simulink model "G_Export_V3"  (R2024b)
settings: Solver=FixedStepDiscrete  StartTime=0  StopTime=1  RelTol=1e-3
libraries: dspxfrm3 x1, dspmlti4 x1, dspsigops x1
settings Model: Creator=Lenovo  LastModifiedBy=Lenovo
settings OptimizationCC: DefaultParameterBehavior=Inlined  EnhancedBackFolding=on  PassReuseOutputArgsAs=Individual arguments  ZeroExternalMemoryAtStartup=off  ZeroInternalMemoryAtStartup=off  OptimizeBlockOrder=speed  DifferentSizesBufferReuse=on  OptimizationCustomize=off  EfficientTunableParamExpr=on
settings DebuggingCC: ParameterTunabilityLossMsg=error
settings HardwareCC: ProdBitPerPointer=32  ProdBitPerSizeT=32  ProdBitPerPtrDiffT=32  ProdLargestAtomicInteger=Long  ProdLargestAtomicFloat=Double  ProdWordSize=32  ProdHWDeviceType=ARM Compatible->ARM Cortex-M
settings SFSimCC: MATLABDynamicMemAlloc=off
settings RTWCC: Description=Embedded Coder  SystemTargetFile=ert.tlc  GenCodeOnly=on  TemplateMakefile=ert_default_tmf
settings CodeAppCC: ForceParamTrailComments=on  GenerateComments=off  IgnoreCustomStorageClasses=off  OperatorAnnotations=on  SimulinkDataObjDesc=on  SFDataObjDesc=on  InsertBlockDesc=on
settings ERTTargetCC: TargetLangStandard=C99 (ISO)  GenerateSampleERTMain=on  SupportNonFinite=off  ERTCustomFileTemplate=example_file_process.tlc

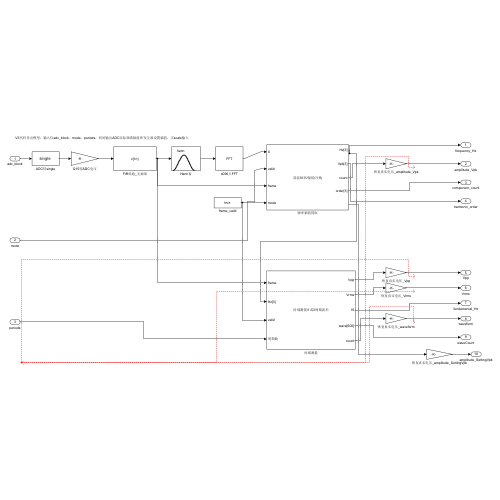
[thumbnail: Simulink's stored preview of the top-level diagram]
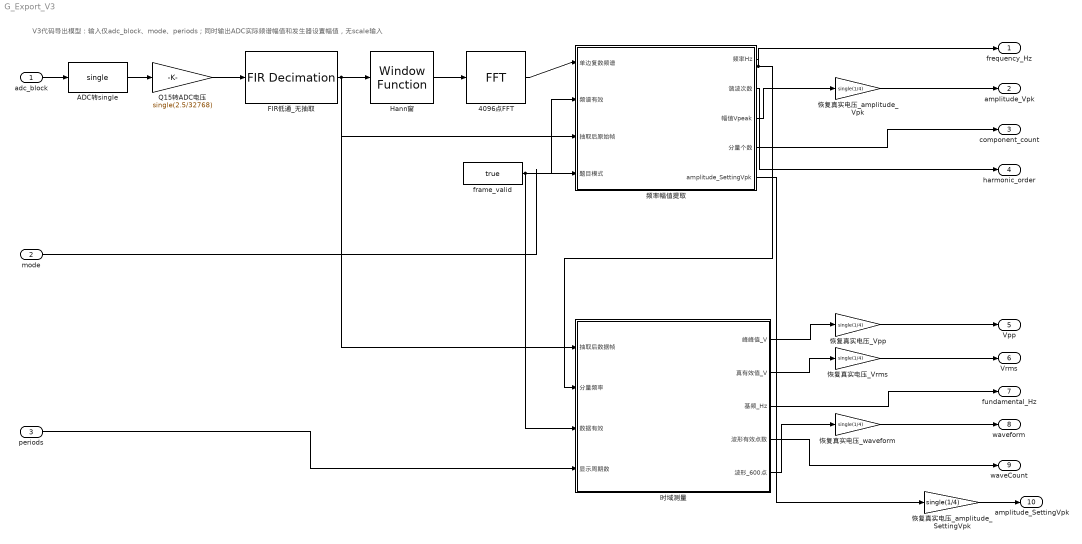
== system G_Export_V3 ==
  note: V3代码导出模型：输入仅adc_block、mode、periods；同时输出ADC实际频谱幅值和发生器设置幅值，无scale输入
  adc_block : Inport  OutDataTypeStr=int16  PortDimensions=16384
  mode : Inport  Port=2  OutDataTypeStr=uint8  PortDimensions=1
  periods : Inport  Port=3  OutDataTypeStr=uint8  PortDimensions=1
  4096点FFT : dspxfrm3/FFT  FFTImplementation=Auto  CompMethod=Table lookup  TableOpt=NEW  TableOptActive=Speed  BitRevOrder=off  Normalize=off  InheritFFTLength=on  FFTLength=64  WrapInput=on  roundingMode=Ceiling  overflowMode=off  firstCoeffDataTypeStr=Inherit: Same word length as input  firstCoeffLastDataTypeStr=Inherit: Same word length as input  outputMin=[]  outputMax=[]
  ADC转single : DataTypeConversion  OutDataTypeStr=single  SaturateOnIntegerOverflow=off  RndMeth=Floor
  FIR低通_无抽取 : dspmlti4/FIR Decimation  FilterSource=Dialog parameters  h=[-1.093832325746845e-05 -6.292254736687438e-05 -0.0001456190566409851 -0.000210121213955772 -0.0001715204318703031 5.201786070564381e-05 0.0004740892277420891 0.0009791364033496543 0.001309961916795507 0.001139443592884425 0.0002271750021134837 -0.001389645221210771 -0.00326542298539904 -0.004577381356277919 -0.004374292500219585 -0.00200400120335077 0.00242713788631572 0.00778010462815952 0.01199664830895183 0.01268492551912718 0.00806980856872996 -0.001995124150862495 -0.01536663043623436 -0.02767001830927002 -0.03323335274731441 -0.02673559895993285 -0.005096036961720372 0.03104031203495614 0.07681183656132551 0.1239468431957101 0.1627378137916923 0.184631371906325 0.184631371906325 0.1627378137916923 0.1239468431957101 0.07681183656132551 0.03104031203495614 -0.005096036961720372 -0.02673559895993285 -0.03323335274731441 -0.02767001830927002 -0.01536663043623436 -0.001995124150862495 0.00806980856872996 0.01268492551912718 0.01199664830895183 0.00778010462815952 0.00242713788631572 -0.00200400120335077 -0.004374292500219585 -0.004577381356277919 -0.00326542298539904 -0.001389645221210771 0.0002271750021134837 0.001139443592884425 0.001309961916795507 0.0009791364033496543 0.0004740892277420891 5.201786070564381e-05 -0.0001715204318703031 -0.000210121213955772 -0.0001456190566409851 -6.292254736687438e-05 -1.093832325746845e-05]  D=1  filtStruct=Direct form transposed  FilterObject=FDECIM  InputProcessing=Columns as channels (frame based)  framing=Enforce single-rate processing  AllowArbitraryInputLength=off  inputOffset=0  outputBufInitCond=0  roundingMode=Floor  overflowMode=off  firstCoeffDataTypeStr=Inherit: Same word length as input  firstCoeffMin=[]  firstCoeffMax=[]  firstCoeffLastDataTypeStr=Inherit: Same word length as input  outputDataTypeStr=Inherit: Same as accumulator  outputMin=[]  outputMax=[]  outputLastDataTypeStr=Inherit: Same as accumulator
  Hann窗 : dspsigops/Window Function  winmode=Apply window to input  wintype=Hann  sampmode=Discrete  samptime=1  N=64  Rs=50  beta=10  winsamp=Symmetric  UserWindow=hamming  OptParams=off  UserParams={'symmetric'}  dataType=double  isSigned=on  wordLen=16  udDataType=sfix(16)  fracBitsMode=Best precision  numFracBits=15  roundingMode=Floor  overflowMode=off  numSidelobes=4  sidelobeLevel=-30
  Q15转ADC电压 : Gain  Gain=single(2.5/32768)
  frame_valid : Constant  Value=true  OutDataTypeStr=boolean
  恢复真实电压_Vpp : Gain  Gain=single(1/4)
  恢复真实电压_Vrms : Gain  Gain=single(1/4)
  恢复真实电压_amplitude_SettingVpk : Gain  Gain=single(1/4)
  恢复真实电压_amplitude_Vpk : Gain  Gain=single(1/4)
  恢复真实电压_waveform : Gain  Gain=single(1/4)
  时域测量 : Subsystem
      mask Display:
      | disp('时域测量/1或3周期波形');
      | port_label('input',1,'frame');
      | port_label('input',2,'Hz[3]');
      | port_label('input',3,'valid');
      | port_label('input',4,'周期数');
      | port_label('output',1,'Vpp');
      | port_label('output',2,'Vrms');
      | port_label('output',3,'f0');
      | port_label('output',4,'wave[600]');
      | port_label('output',5,'count');
  频率幅值提取 : Subsystem  mask{Fs=8e6, NFFT=16384, MinFreq=10e3, MaxFreq=500e3, MinAmp=4e-3}
      mask prompts: Fs "采样率 Fs (Hz)"; NFFT "FFT点数 NFFT"; MinFreq "最低分析频率 (Hz)"; MaxFreq "最高分析频率 (Hz)"; MinAmp "最小有效幅值 (Vpeak)"
      mask Display:
      | disp('谐波频率/幅值/次数');
      | port_label('input',1,'X');
      | port_label('input',2,'valid');
      | port_label('input',3,'frame');
      | port_label('input',4,'mode');
      | port_label('output',1,'Hz[3]');
      | port_label('output',2,'Vpk[3]');
      | port_label('output',3,'count');
      | port_label('output',4,'order[3]');
  frequency_Hz : Outport
  amplitude_Vpk : Outport  Port=2
  component_count : Outport  Port=3
  harmonic_order : Outport  Port=4
  Vpp : Outport  Port=5
  Vrms : Outport  Port=6
  fundamental_Hz : Outport  Port=7
  waveform : Outport  Port=8
  waveCount : Outport  Port=9
  amplitude_SettingVpk : Outport  Port=10
  wires:
  adc_block/1 -> ADC转single/1
  ADC转single/1 -> Q15转ADC电压/1
  Q15转ADC电压/1 -> FIR低通_无抽取/1
  FIR低通_无抽取/1 -> Hann窗/1, 频率幅值提取/3(抽取后原始帧), 时域测量/1(抽取后数据帧)
  Hann窗/1 -> 4096点FFT/1
  4096点FFT/1 -> 频率幅值提取/1(单边复数频谱)
  frame_valid/1 -> 频率幅值提取/2(频谱有效), 时域测量/3(数据有效)
  mode/1 -> 频率幅值提取/4(题目模式)
  频率幅值提取/1(频率Hz) -> 时域测量/2(分量频率), frequency_Hz/1
  periods/1 -> 时域测量/4(显示周期数)
  频率幅值提取/3(幅值Vpeak) -> 恢复真实电压_amplitude_Vpk/1
  ? -> ?
  频率幅值提取/4(分量个数) -> component_count/1
  频率幅值提取/2(谐波次数) -> harmonic_order/1
  时域测量/1(峰峰值_V) -> 恢复真实电压_Vpp/1
  时域测量/2(真有效值_V) -> 恢复真实电压_Vrms/1
  时域测量/3(基频_Hz) -> fundamental_Hz/1
  时域测量/5(波形_600点) -> 恢复真实电压_waveform/1
  时域测量/4(波形有效点数) -> waveCount/1
  恢复真实电压_Vpp/1 -> Vpp/1
  恢复真实电压_Vrms/1 -> Vrms/1
  恢复真实电压_amplitude_Vpk/1 -> amplitude_Vpk/1
  恢复真实电压_waveform/1 -> waveform/1
  频率幅值提取/5(amplitude_SettingVpk) -> 恢复真实电压_amplitude_SettingVpk/1
  恢复真实电压_amplitude_SettingVpk/1 -> amplitude_SettingVpk/1

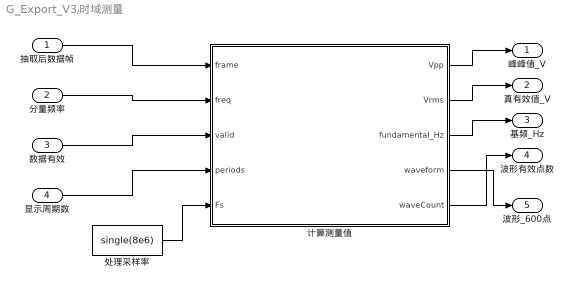
== system G_Export_V3/时域测量 ==
  抽取后数据帧 : Inport
  分量频率 : Inport  Port=2
  数据有效 : Inport  Port=3
  显示周期数 : Inport  Port=4
  处理采样率 : Constant  Value=single(8e6)  OutDataTypeStr=single
  计算测量值 : MATLAB Function  TreatAsAtomicUnit=on
  峰峰值_V : Outport
  真有效值_V : Outport  Port=2
  基频_Hz : Outport  Port=3
  波形有效点数 : Outport  Port=4
  波形_600点 : Outport  Port=5
  wires:
  计算测量值/5(waveCount) -> 波形有效点数/1
  计算测量值/4(waveform) -> 波形_600点/1
  计算测量值/3(fundamental_Hz) -> 基频_Hz/1
  计算测量值/2(Vrms) -> 真有效值_V/1
  计算测量值/1(Vpp) -> 峰峰值_V/1
  处理采样率/1 -> 计算测量值/5(Fs)
  显示周期数/1 -> 计算测量值/4(periods)
  数据有效/1 -> 计算测量值/3(valid)
  分量频率/1 -> 计算测量值/2(freq)
  抽取后数据帧/1 -> 计算测量值/1(frame)

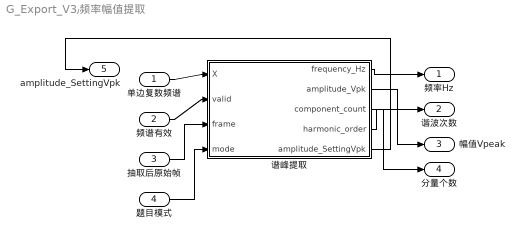
== system G_Export_V3/频率幅值提取 ==
  单边复数频谱 : Inport
  频谱有效 : Inport  Port=2
  抽取后原始帧 : Inport  Port=3
  题目模式 : Inport  Port=4
  谱峰提取 : MATLAB Function  TreatAsAtomicUnit=on
  频率Hz : Outport
  谐波次数 : Outport  Port=2
  幅值Vpeak : Outport  Port=3
  分量个数 : Outport  Port=4
  amplitude_SettingVpk : Outport  Port=5
  wires:
  谱峰提取/4(harmonic_order) -> 谐波次数/1
  题目模式/1 -> 谱峰提取/4(mode)
  抽取后原始帧/1 -> 谱峰提取/3(frame)
  谱峰提取/3(component_count) -> 分量个数/1
  谱峰提取/2(amplitude_Vpk) -> 幅值Vpeak/1
  谱峰提取/1(frequency_Hz) -> 频率Hz/1
  频谱有效/1 -> 谱峰提取/2(valid)
  单边复数频谱/1 -> 谱峰提取/1(X)
  谱峰提取/5(amplitude_SettingVpk) -> amplitude_SettingVpk/1

== matlab function G_Export_V3/频率幅值提取/谱峰提取 ==
  data: X input; frequency_Hz output; valid input; frame input; mode input; amplitude_Vpk output; component_count output; Fs parameter; NFFT parameter; MinFreq parameter; MaxFreq parameter; MinAmp parameter; harmonic_order output; amplitude_SettingVpk output
function [frequency_Hz, amplitude_Vpk, component_count, harmonic_order, amplitude_SettingVpk] = fcn(X, valid, frame, mode, Fs, NFFT, MinFreq, MaxFreq, MinAmp)
%#codegen
N=coder.const(NFFT);
frequency_Hz=zeros(3,1,'single');
amplitude_Vpk=zeros(3,1,'single');
amplitude_SettingVpk=zeros(3,1,'single');
component_count=uint8(0);
harmonic_order=zeros(3,1,'uint8');
if ~valid
    return;
end
mag=abs(X);
k0=max(2,ceil(MinFreq*N/Fs)+1);
if mode==1
    maxF=single(200e3);
else
    maxF=single(500e3);
end
k1=min(N/2,ceil(double(maxF)*N/Fs)+2);
bestScore=zeros(3,1,'single');
bestBin=zeros(3,1,'single');
for k=k0:k1
    if mag(k)>=mag(k-1) && mag(k)>mag(k+1)
        y1=log(max(mag(k-1),single(1e-30)));
        y2=log(max(mag(k),single(1e-30)));
        y3=log(max(mag(k+1),single(1e-30)));
        den=y1-2*y2+y3;
        delta=single(0);
        if abs(den)>single(1e-20)
            delta=single(0.5)*(y1-y3)/den;
        end
        delta=min(single(0.5),max(single(-0.5),delta));
        ampApprox=single(2)*(mag(k-1)+mag(k)+mag(k+1))/single(N-1);
        if ampApprox>=single(MinAmp)
            for j=1:3
                if ampApprox>bestScore(j)
                    for q=3:-1:j+1
                        bestScore(q)=bestScore(q-1); bestBin(q)=bestBin(q-1);
                    end
                    bestScore(j)=ampApprox; bestBin(j)=single(k-1)+delta;
                    break;
                end
            end
        end
    end
end
for j=1:3
    if bestScore(j)>0
        frequency_Hz(j)=bestBin(j)*single(Fs/N);
        component_count=component_count+1;
    end
end
for a=1:2
    for bidx=a+1:3
        if frequency_Hz(bidx)>0 && (frequency_Hz(a)==0 || frequency_Hz(bidx)<frequency_Hz(a))
            tf=frequency_Hz(a); frequency_Hz(a)=frequency_Hz(bidx); frequency_Hz(bidx)=tf;
        end
    end
end
if frequency_Hz(1)>0
    for j=1:3
        if frequency_Hz(j)>0
            ratio=frequency_Hz(j)/frequency_Hz(1);
            orderValue=round(ratio);
            if orderValue>=1 && orderValue<=255 && abs(ratio-orderValue)<single(0.15)
                harmonic_order(j)=uint8(orderValue);
            end
        end
    end
end
dc=single(0);
for n=1:N
    dc=dc+frame(n);
end
dc=dc/single(N);
% Estimate the repeated waveform peak robustly.  A single maximum
% is too sensitive to ADC noise or an isolated repaired sample.
rawPeakAbs=single(0);
for n=1:N
    ay=abs(frame(n)-dc);
    if ay>rawPeakAbs
        rawPeakAbs=ay;
    end
end
peakThreshold=rawPeakAbs*single(0.99);
peakSum=single(0);
peakCount=uint32(0);
for n=2:N-1
    ym=abs(frame(n-1)-dc);
    y0=abs(frame(n)-dc);
    yp=abs(frame(n+1)-dc);
    if y0>=peakThreshold && y0>=ym && y0>yp
        peakSum=peakSum+y0;
        peakCount=peakCount+uint32(1);
    end
end
framePeakAbs=rawPeakAbs;
if peakCount>uint32(0)
    framePeakAbs=peakSum/single(peakCount);
end
for j=1:3
    f=frequency_Hz(j);
    if f>0
        omega=single(2*pi)*f/single(Fs);
        cw=cos(omega); sw=sin(omega);
        c=single(1); s=single(0);
        cc=single(0); ss=single(0); cs=single(0); yc=single(0); ys=single(0);
        for n=1:N
            y=frame(n)-dc;
            cc=cc+c*c; ss=ss+s*s; cs=cs+c*s;
            yc=yc+y*c; ys=ys+y*s;
            cn=c*cw-s*sw; sn=s*cw+c*sw; c=cn; s=sn;
            if bitand(n,255)==0
                r=sqrt(c*c+s*s); c=c/r; s=s/r;
            end
        end
        detv=cc*ss-cs*cs;
        if abs(detv)>single(1e-20)
            ac=(yc*ss-ys*cs)/detv;
            as=(ys*cc-yc*cs)/detv;
            amplitude_Vpk(j)=sqrt(ac*ac+as*as);
        end
    end
end
correction=single(1);
if amplitude_Vpk(1)>single(1e-6) && framePeakAbs>amplitude_Vpk(1)*single(1.005)
    correction=framePeakAbs/amplitude_Vpk(1);
end
for j=1:3
    amplitude_SettingVpk(j)=amplitude_Vpk(j)*correction;
end
end

== matlab function G_Export_V3/时域测量/计算测量值 ==
  data: frame input; Vpp output; freq input; valid input; periods input; Fs input; Vrms output; fundamental_Hz output; waveform output; waveCount output
function [Vpp, Vrms, fundamental_Hz, waveform, waveCount] = fcn(frame, freq, valid, periods, Fs)
%#codegen
MAX_POINTS = 600;
waveform = zeros(MAX_POINTS,1,'single');
Vpp = single(0);
Vrms = single(0);
fundamental_Hz = single(0);
waveCount = uint16(0);
if ~valid
    return;
end
N = numel(frame);
dc = single(0);
for n = 1:N
    dc = dc + frame(n);
end
dc = dc / single(N);
energy = single(0);
imax = 1;
imin = 1;
ymax = frame(1) - dc;
ymin = ymax;
for n = 1:N
    y = frame(n) - dc;
    energy = energy + y*y;
    if y > ymax
        ymax = y; imax = n;
    end
    if y < ymin
        ymin = y; imin = n;
    end
end
Vrms = sqrt(energy / single(N));
ymax = peak_vertex(frame, dc, imax, N, true);
ymin = peak_vertex(frame, dc, imin, N, false);
Vpp = ymax - ymin;
fundamental_Hz = freq(1);
if fundamental_Hz <= 0
    return;
end
p = 1;
if periods >= 3
    p = 3;
end
samplesPerPeriod = single(Fs) / fundamental_Hz;
span = single(p) * samplesPerPeriod;
required = ceil(double(span)) + 2;
if required >= N
    return;
end
startIndex = 1;
lastStart = N - required;
for n = 2:lastStart
    if frame(n-1)-dc <= 0 && frame(n)-dc > 0
        startIndex = n;
        break;
    end
end
for n = 1:MAX_POINTS
    pos = single(startIndex) + single(n-1)*span/single(MAX_POINTS-1);
    i0 = floor(double(pos));
    frac = pos - single(i0);
    if i0 < 1
        i0 = 1; frac = single(0);
    elseif i0 >= N
        i0 = N-1; frac = single(1);
    end
    y0 = frame(i0) - dc;
    y1 = frame(i0+1) - dc;
    waveform(n) = y0 + frac*(y1-y0);
end
waveCount = uint16(MAX_POINTS);
end

function yv = peak_vertex(x, dc, k, N, isMaximum)
%#codegen
km = k-1; if km < 1, km = N; end
kp = k+1; if kp > N, kp = 1; end
ym = x(km)-dc; y0 = x(k)-dc; yp = x(kp)-dc;
den = single(8)*(yp+ym-single(2)*y0);
yv = y0;
if abs(den) > single(1e-12)
    candidate = y0 - (yp-ym)*(yp-ym)/den;
    if (isMaximum && candidate >= y0) || (~isMaximum && candidate <= y0)
        yv = candidate;
    end
end
end
